simulink model "calculator"  (R2021a)
settings: Solver=FixedStepDiscrete  StartTime=0.0  StopTime=10.0  RelTol=1e-3  EnableMultiTasking=on
libraries: simulink x3
settings Model: Creator=iT-User  LastModifiedBy=iT-User
settings DataIOCC: ReturnWorkspaceOutputs=off
settings OptimizationCC: DefaultParameterBehavior=Inlined  InlineInvariantSignals=on  EnableMemcpy=off  LifeSpan=1  EfficientTunableParamExpr=on
settings DebuggingCC: UnderspecifiedInitializationDetection=Classic  MergeDetectMultiDrivingBlocksExec=none  SFMachineParentedDataDiag=warning  ArithmeticOperatorsInVariantConditions=warning
settings ModelReferenceCC: PropagateSignalLabelsOutOfModel=off
settings SFSimCC: MATLABDynamicMemAlloc=off  CustomCodeUndefinedFunction=UseInterfaceOnly
settings RTWCC: SystemTargetFile=ert.tlc  GenCodeOnly=on  TemplateMakefile=ert_default_tmf  GenerateReport=on  IncludeHyperlinkInReport=on  LaunchReport=on  GenerateTraceInfo=on  GenerateTraceReport=on  GenerateTraceReportSl=on  GenerateTraceReportSf=on  GenerateTraceReportEml=on
settings CodeAppCC: ForceParamTrailComments=on  IgnoreCustomStorageClasses=off  OperatorAnnotations=on  SimulinkDataObjDesc=on  SFDataObjDesc=on  MATLABFcnDesc=on  InsertBlockDesc=on  StateflowObjectComments=on  MATLABSourceComments=on
settings ERTTargetCC: MultiwordLength=2048  GenerateSampleERTMain=on  InlinedParameterPlacement=NonHierarchical  ERTCustomFileTemplate=example_file_process.tlc

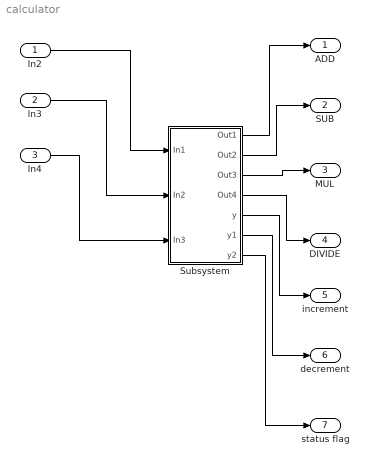
== system calculator ==
  In2 : Inport
  In3 : Inport  Port=2
  In4 : Inport  Port=3
  Subsystem : Subsystem
  ADD : Outport
  SUB : Outport  Port=2
  MUL : Outport  Port=3
  DIVIDE : Outport  Port=4
  increment : Outport  Port=5
  decrement : Outport  Port=6
  status flag : Outport  Port=7
  wires:
  In2/1 -> Subsystem/1(In1)
  In3/1 -> Subsystem/2(In2)
  In4/1 -> Subsystem/3(In3)
  Subsystem/1(Out1) -> ADD/1
  Subsystem/2(Out2) -> SUB/1
  Subsystem/3(Out3) -> MUL/1
  Subsystem/4(Out4) -> DIVIDE/1
  Subsystem/5(y) -> increment/1
  Subsystem/6(y1) -> decrement/1
  Subsystem/7(y2) -> status flag/1

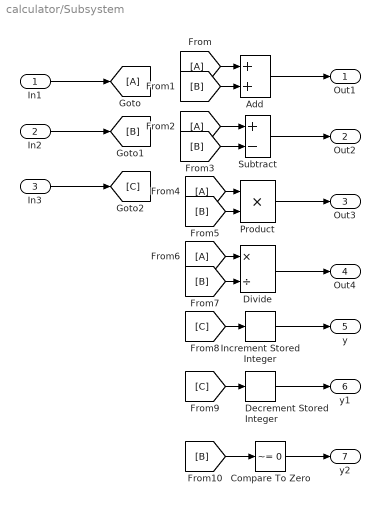
== system calculator/Subsystem ==
  In1 : Inport
  In2 : Inport  Port=2
  In3 : Inport  Port=3
  Add : Sum
  Compare To Zero : simulink/Logic and Bit Operations/Compare To Zero  relop=~=  OutDataTypeStr=uint8
  Decrement Stored Integer : simulink/Additional Math & Discrete/Additional Math: Increment - Decrement/Decrement Stored Integer
      settings: SourceProductBaseCode=SL
  Divide : Product  Inputs=*/
  Increment Stored Integer : simulink/Additional Math & Discrete/Additional Math: Increment - Decrement/Increment Stored Integer
  Product : Product
  Subtract : Sum  Inputs=+-
  Out1 : Outport
  Out2 : Outport  Port=2
  Out3 : Outport  Port=3
  Out4 : Outport  Port=4
  y : Outport  Port=5
  y1 : Outport  Port=6
  y2 : Outport  Port=7
  wires:
  [C] -> Increment Stored Integer/1
  [A] -> Subtract/1
  [A] -> Product/1
  [C] -> Decrement Stored Integer/1
  Increment Stored Integer/1 -> y/1
  [B] -> Product/2
  [B] -> Divide/2
  [B] -> Compare To Zero/1
  Subtract/1 -> Out2/1
  [A] -> Add/1
  [A] -> Divide/1
  [B] -> Subtract/2
  In2/1 -> [B]
  [B] -> Add/2
  Decrement Stored Integer/1 -> y1/1
  In1/1 -> [A]
  Compare To Zero/1 -> y2/1
  Divide/1 -> Out4/1
  Product/1 -> Out3/1
  Add/1 -> Out1/1
  In3/1 -> [C]
